simulink model "comp4bit"  (R2020a)
settings: Solver=VariableStepAuto  StartTime=0.0  StopTime=10.0  RelTol=1e-3
settings Model: Creator=kishan  LastModifiedBy=kishan

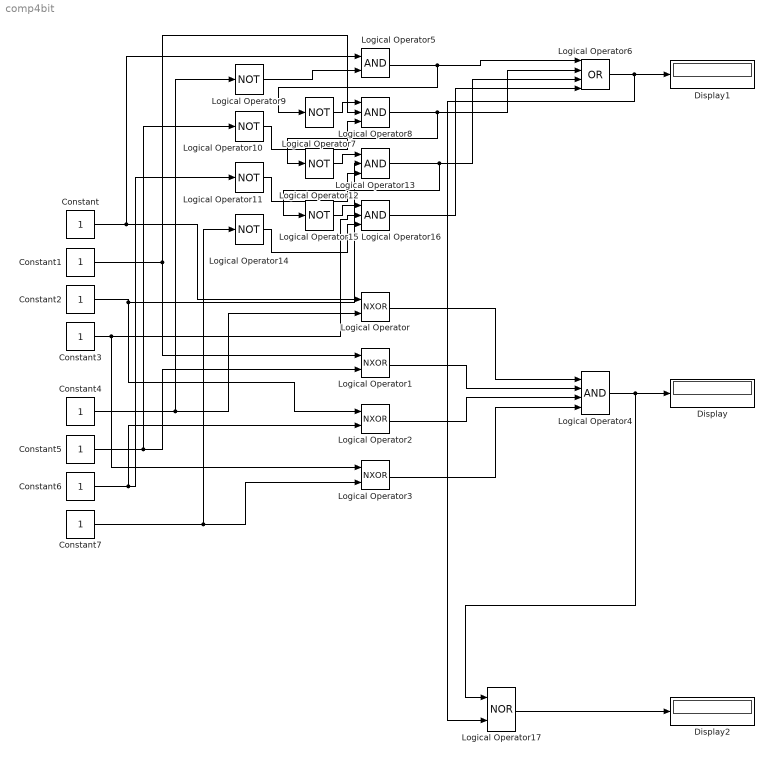
== system comp4bit ==
  Constant{,1..7} (8 alike) : Constant
  Display : Display
  Display1 : Display
  Display2 : Display
  Logical Operator{,1..3} (4 alike) : Logic  Operator=NXOR  AllPortsSameDT=off  OutDataTypeStr=boolean
  Logical Operator{7,9..12,14..15} (7 alike) : Logic  Operator=NOT  Inputs=3  AllPortsSameDT=off  OutDataTypeStr=boolean
  Logical Operator13 : Logic  Inputs=3  AllPortsSameDT=off  OutDataTypeStr=boolean
  Logical Operator16 : Logic  Inputs=3  AllPortsSameDT=off  OutDataTypeStr=boolean
  Logical Operator17 : Logic  Operator=NOR  AllPortsSameDT=off  OutDataTypeStr=boolean
  Logical Operator4 : Logic  Inputs=4  AllPortsSameDT=off  OutDataTypeStr=boolean
  Logical Operator5 : Logic  AllPortsSameDT=off  OutDataTypeStr=boolean
  Logical Operator6 : Logic  Operator=OR  Inputs=4  AllPortsSameDT=off  OutDataTypeStr=boolean
  Logical Operator8 : Logic  Inputs=3  AllPortsSameDT=off  OutDataTypeStr=boolean
  wires:
  Constant/1 -> Logical Operator5/1, Logical Operator/1
  Constant4/1 -> Logical Operator9/1, Logical Operator/2
  Constant1/1 -> Logical Operator8/2, Logical Operator1/1
  Constant5/1 -> Logical Operator10/1, Logical Operator1/2
  Constant2/1 -> Logical Operator13/2, Logical Operator2/1
  Constant3/1 -> Logical Operator16/2, Logical Operator3/1
  Constant7/1 -> Logical Operator14/1, Logical Operator3/2
  Logical Operator/1 -> Logical Operator4/1
  Logical Operator1/1 -> Logical Operator4/2
  Logical Operator2/1 -> Logical Operator4/3
  Logical Operator3/1 -> Logical Operator4/4
  Logical Operator4/1 -> Logical Operator17/1, Display/1
  Constant6/1 -> Logical Operator11/1, Logical Operator2/2
  Logical Operator9/1 -> Logical Operator5/2
  Logical Operator6/1 -> Logical Operator17/2, Display1/1
  Logical Operator5/1 -> Logical Operator7/1, Logical Operator6/1
  Logical Operator8/1 -> Logical Operator12/1, Logical Operator6/2
  Logical Operator10/1 -> Logical Operator8/3
  Logical Operator7/1 -> Logical Operator8/1
  Logical Operator11/1 -> Logical Operator13/3
  Logical Operator12/1 -> Logical Operator13/1
  Logical Operator14/1 -> Logical Operator16/3
  Logical Operator15/1 -> Logical Operator16/1
  Logical Operator13/1 -> Logical Operator15/1, Logical Operator6/3
  Logical Operator16/1 -> Logical Operator6/4
  Logical Operator17/1 -> Display2/1
